simulink library "hose_pump_unit_v4"  (R2025b)
settings: Solver=VariableStepAuto  StartTime=0.0  StopTime=10.0  RelTol=1e-3
undefined symbols (not defined in the file): ACV_fit_coeffs, HP_bladder_elastic_modulus, HP_flowrate_damping_coefficient, HP_unstretched_fiber_angle, HP_unstretched_length, HP_unstretched_radius, HP_unstretched_wall_thickness, L_inlet, mu, power_avg_start_time, PTO_capacity_W, R_inlet, regulator_set_pressure_PSI, simu, SV_closing_threshold_Pa, SV_opening_threshold_Pa, turbine_gear_ratio
libraries: simulink x28, dspstat3 x4, turbine_generator_v0 x2, dsppolyfun x1, adjustable_check_valve_v0 x1
(part 1 of 2)
settings Model: Creator=Carson  LastModifiedBy=cmmcguir

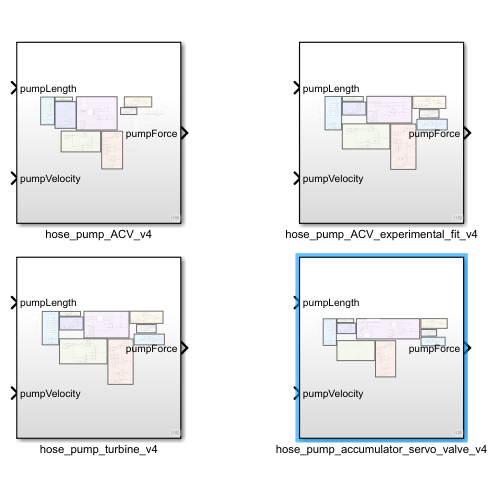
[thumbnail: Simulink's stored preview of the top-level diagram]
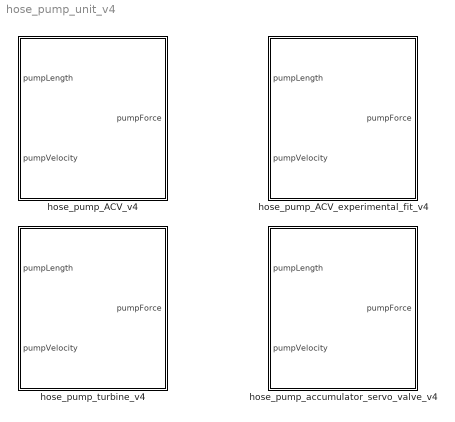
== system hose_pump_unit_v4 ==
  hose_pump_ACV_experimental_fit_v4 : Subsystem
  hose_pump_ACV_v4 : Subsystem
  hose_pump_accumulator_servo_valve_v4 : Subsystem
  hose_pump_turbine_v4 : Subsystem

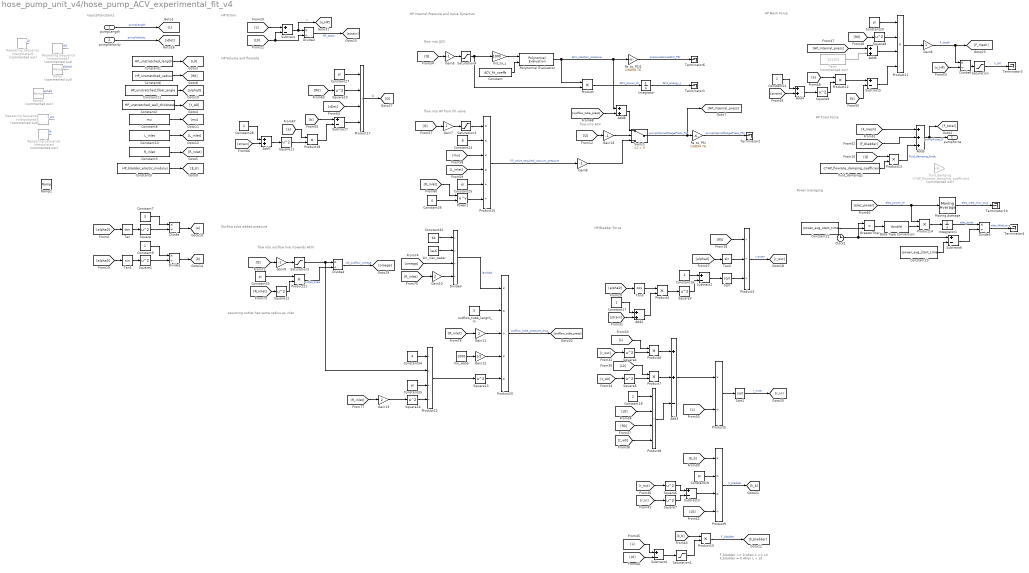
== system hose_pump_unit_v4/hose_pump_ACV_experimental_fit_v4 ==
  note: flow into ACV
  note: flow into ACV
  note: F_bladder >= 0 when L >= L0
      | F_bladder = 0 when L < L0
  note: HP Total Force
  note: HP Mesh Force
  note: HP Bladder Force
  note: HP Internal Pressure and Valve Dynamics
  note: HP Strain
  note: HP Volume and flowrate
  note: Inputs/Constants
  note: flow into HP from fill valve
  note: flow into outflow line (towards ACV)
  note: assuming outlet has same radius as inlet
  note: Outflow tube added pressure
  note: Power averaging
  pumpLength : Inport
  pumpVelocity : Inport  Port=2
  Add{2,4,6..8} (5 alike) : Sum
  Add3 : Sum  Inputs=++-
  Add5 : Sum  Inputs=+++
  Clock1 : Clock
  Constant : Constant  Value=ACV_fit_coeffs
  Constant1 : Constant  Value=HP_unstretched_length
  Constant10 : Constant  Value=L_inlet
  Constant11 : Constant  Value=HP_unstretched_fiber_angle
  Constant{9,16..17,21,28} (5 alike) : Constant
  Constant18 : Constant  Value=2
  Constant{19..20,25,27,33,35} (6 alike) : Constant  Value=pi
  Constant2 : Constant  Value=HP_unstretched_wall_thickness
  Constant22 : Constant  Value=power_avg_start_time
  Constant23 : Constant  Value=power_avg_start_time
  Constant24 : Constant  Value=8
  Constant26 : Constant  Value=4
  Constant3 : Constant  Value=R_inlet
  Constant32 : Constant  Value=64
  Constant34 : Constant  Value=4
  Constant5 : Constant  Value=HP_bladder_elastic_modulus
  Constant6 : Constant  Value=HP_unstretched_radius
  Constant7 : Constant  Value=3
  Constant8 : Constant  Value=mu
  Data Type Conversion : DataTypeConversion  OutDataTypeStr=double  SaturateOnIntegerOverflow=off  RndMeth=Floor
  Divide{,1..2,4..6} (6 alike) : Product  Inputs=*/
  Divide3 : Product  Inputs=**//
  Gain10 : Gain  Gain=2
  Gain11 : Gain  Gain=2
  Gain12 : Gain  Gain=1/2
  Gain13 : Gain  Gain=2
  Gain{5,8..9,14} (4 alike) : Gain  Gain=-1
  Gain6 : Gain
  Gain7 : Gain
  GreaterThan : RelationalOperator  Operator=>  OutDataTypeStr=boolean  RndMeth=Simplest  InputSameDT=off
  Integrator : Integrator
  Integrator1 : Integrator
  Moving Average : dspstat3/Moving Average  Method=Sliding window  ForgettingFactorPort=off  SpecifyWindowLength=on  WindowLength=30 / simu.dt  OverlapLength=30 / simu.dt - 1  AllowArbitraryInputLength=off  ForgettingFactor=0.9  SimulateUsing=Interpreted execution
  Pa_to_PSI : Gain  Gain=1/6894.76
  Pa_to_PSI1 : Gain  Gain=1/6894.76
  Patm : Constant  Commented=on  Value=101325
  Polynomial Evaluation : dsppolyfun/Polynomial Evaluation  useConstCoeffs=off  constCoeffs=[5 4 3 2 1]
  Power1 : Math  Operator=pow
  Product{,4,6..7,10,12..14,18,21} (10 alike) : Product
  Product11 : Product  Inputs=****
  Product15 : Product  Inputs=****//
  Product17 : Product  Inputs=****
  Product20 : Product  Inputs=**/**
  Product22 : Product  Inputs=**//
  Product3 : Product  Inputs=*/*
  Product5 : Product  Inputs=*/
  Product8 : Product  Inputs=****
  Product9 : Product  Inputs=***/
  Ramp : simulink/Sources/Ramp  Commented=on  slope=(1.25-1.12) / 2400  start=30  InitialOutput=1.12
  Ramp1 : simulink/Sources/Ramp  slope=5/1200  start=30  InitialOutput=1
  Ramp2 : simulink/Sources/Ramp  Commented=on  slope=(1.1 - 0.9) * HP_unstretched_fiber_angle / 2400  start=30  InitialOutput=0.9 * HP_unstretched_fiber_angle
  Repeating Sequence Interpolated : simulink/Sources/Repeating Sequence Interpolated  Commented=on  OutValues=HP_bladder_elastic_modulus * [0.75 2 0.75]  TimeValues=[0 60 120]*2  LookUpMeth=Interpolation-Use End Values  tsamp=simu.dt  OutMin=[]  OutMax=[]  OutDataTypeStr=double  OutputDataTypeScalingMode=double  OutDataType=fixdt(0,8)  OutScaling=2^-10
  Repeating Sequence Interpolated1 : simulink/Sources/Repeating Sequence Interpolated  Commented=on  OutValues=HP_unstretched_length * [0.8 1.2 0.8]  TimeValues=[0 60 120] * 4  LookUpMeth=Interpolation-Use End Values  tsamp=simu.dt  OutMin=[]  OutMax=[]  OutDataTypeStr=double  OutputDataTypeScalingMode=double  OutDataType=fixdt(0,8)  OutScaling=2^-10
  Repeating Sequence Interpolated2 : simulink/Sources/Repeating Sequence Interpolated  Commented=on  OutValues=HP_unstretched_radius * [0.8 1.2 0.8]  TimeValues=[0 60 120] * 4  LookUpMeth=Interpolation-Use End Values  tsamp=simu.dt  OutMin=[]  OutMax=[]  OutDataTypeStr=double  OutputDataTypeScalingMode=double  OutDataType=fixdt(0,8)  OutScaling=2^-10
  Repeating Sequence Interpolated3 : simulink/Sources/Repeating Sequence Interpolated  Commented=on  OutValues=HP_unstretched_wall_thickness * [0.75 1.25 0.75]  TimeValues=[0 60 120] * 4  LookUpMeth=Interpolation-Use End Values  tsamp=simu.dt  OutMin=[]  OutMax=[]  OutDataTypeStr=double  OutputDataTypeScalingMode=double  OutDataType=fixdt(0,8)  OutScaling=2^-10
  Saturation : Saturate  UpperLimit=10000  LowerLimit=-10000
  Saturation1 : Saturate  UpperLimit=inf  LowerLimit=0
  Saturation3 : Saturate  UpperLimit=inf  LowerLimit=0
  Saturation4 : Saturate  UpperLimit=inf  LowerLimit=0
  Saturation5 : Saturate  UpperLimit=inf  LowerLimit=1e-8
  Sqrt : Sqrt
  Sqrt1 : Sqrt
  Square{,1,3..14} (14 alike) : Math  Operator=square
  Subtract{,2..7} (7 alike) : Sum  Inputs=+-
  Switch : Switch  Criteria=u2 > Threshold  SaturateOnIntegerOverflow=off  InputSameDT=off
  Tan : Trigonometry  Operator=tan
  Tan1 : Trigonometry
  Tan2 : Trigonometry
  Tan3 : Trigonometry  Operator=cos
  Terminator{1..4,6,10} (6 alike) : Terminator
  fluid_damping : Gain  Commented=on  Gain=-1*HP_flowrate_damping_coefficient
  fluid_damping1 : Constant  Value=-1*HP_flowrate_damping_coefficient
  kin_visc_water : Constant  Value=1e-6
  m3_to_L : Gain  Gain=1000
  outflow_tube_length_m : Constant  Value=3
  rho_water : Constant  Value=1000
  pumpForce : Outport
  wires:
  [Q] -> Gain14/1
  [outflow_tube_press] -> Add8/2
  Constant2/1 -> [t_w0]
  Constant1/1 -> [L0]
  Constant5/1 -> [E_b]
  Constant11/1 -> [alpha0]
  pumpLength/1 -> [L]  "pumpLength"
  Constant6/1 -> [R0]
  Constant8/1 -> [mu]
  Constant10/1 -> [L_inlet]
  Switch/1 -> [HP_internal_press], Pa_to_PSI/1  "pumpInternalGuagePress_Pa"
  Pa_to_PSI/1 -> Terminator2/1  "pumpInternalGuagePress_PSI"
  Constant3/1 -> [R_inlet]
  Constant7/1 -> Divide/1
  [alpha0] -> Tan/1
  Tan/1 -> Square/1
  Square/1 -> Divide/2
  Divide/1 -> [a]
  Divide1/1 -> [b]
  Square1/1 -> Divide1/2
  Tan1/1 -> Square1/1
  [alpha0] -> Tan1/1
  Constant9/1 -> Divide1/1
  [L] -> Subtract/1
  [L0] -> Divide2/2, Subtract/2
  Subtract/1 -> [x_HP], Divide2/1  "x"
  Divide2/1 -> [strain]  "HP_strain"
  [R0] -> Product3/1
  [alpha0] -> Tan2/1
  Tan2/1 -> Product3/2
  Sqrt/1 -> Product3/3
  Subtract2/1 -> Sqrt/1
  Constant16/1 -> Subtract2/1
  [alpha0] -> Tan3/1
  Square3/1 -> Subtract2/2
  Product4/1 -> Square3/1
  Tan3/1 -> Product4/1
  Constant17/1 -> Add2/1
  [strain] -> Add2/2
  Add2/1 -> Product4/2
  Product3/1 -> [r_out]  "r_outer"
  Sqrt1/1 -> [r_in]  "r_inner"
  Product5/1 -> Sqrt1/1
  [L] -> Product5/2
  Add3/1 -> Product5/1
  Product6/1 -> Add3/1
  Square4/1 -> Product6/2
  [r_out] -> Square4/1
  [L] -> Product6/1
  [L0] -> Product7/1
  [t_w0] -> Square5/1
  Square5/1 -> Product7/2
  Product7/1 -> Add3/2
  Product8/1 -> Add3/3
  Constant18/1 -> Product8/1
  [L0] -> Product8/2
  [R0] -> Product8/3
  [t_w0] -> Product8/4
  [E_b] -> Product9/1
  Constant19/1 -> Product9/2
  Subtract3/1 -> Product9/3
  [r_out] -> Square6/1
  Square6/1 -> Subtract3/1
  [r_in] -> Square7/1
  Square7/1 -> Subtract3/2
  [L0] -> Product9/4
  Product9/1 -> [k_b]  "k_bladder"
  [k_b] -> Product10/1
  Subtract4/1 -> Saturation1/1
  [L0] -> Subtract4/2
  [L] -> Subtract4/1
  Product10/1 -> [F_bladder]  "F_bladder"
  [R0] -> Square8/1
  Constant20/1 -> Product11/1
  Square8/1 -> Product11/2
  [HP_internal_press] -> Add6/1
  [a] -> Product12/1
  Constant21/1 -> Add4/1
  Add4/1 -> Square9/1
  [strain] -> Add4/2
  Square9/1 -> Product12/2
  Product12/1 -> Subtract5/1
  [b] -> Subtract5/2
  Subtract5/1 -> Product11/4
  Gain6/1 -> Divide6/1, [F_mesh]  "F_mesh"
  Product13/1 -> Add5/3  "fluid_damping_force"
  Add5/1 -> [F_total], pumpForce/1  "pumpForce_N"
  Patm/1 -> Add6/2
  Add6/1 -> Product11/3
  [elec_power] -> Moving Average/1, Product14/1  "elec_power_W"
  Integrator1/1 -> Divide5/1  "elec_Joule"
  Divide5/1 -> Terminator4/1  "elec_Watt_avg"
  GreaterThan/1 -> Data Type Conversion/1
  Subtract6/1 -> Divide5/2
  Product14/1 -> Integrator1/1
  Constant23/1 -> Subtract6/2
  Constant22/1 -> GreaterThan/2
  Data Type Conversion/1 -> Product14/2
  Clock1/1 -> GreaterThan/1, Subtract6/1
  Saturation1/1 -> Product10/2
  [Q] -> Gain5/1
  Polynomial Evaluation/1 -> Product/1, Pa_to_PSI1/1, Add8/1  "ACV_reaction_pressure"
  [Q] -> Gain7/1
  Gain7/1 -> Saturation3/1
  Saturation3/1 -> Product15/1
  Constant24/1 -> Product15/2
  [mu] -> Product15/3
  [L_inlet] -> Product15/4
  Constant25/1 -> Product15/5
  Power1/1 -> Product15/6
  [R_inlet] -> Power1/1
  Constant26/1 -> Power1/2
  Product15/1 -> Gain8/1  "fill_valve_required_vacuum_pressure"
  Gain8/1 -> Switch/3
  Saturation4/1 -> Product/2, m3_to_L/1
  [F_mesh] -> Add5/1
  [F_bladder] -> Add5/2
  pumpVelocity/1 -> [xDot]  "pumpVelocity"
  Product17/1 -> [Q]  "Q"
  Square10/1 -> Product17/2
  Constant27/1 -> Product17/1
  [R0] -> Square10/1
  [xDot] -> Product17/3
  Subtract7/1 -> Product17/4
  [b] -> Subtract7/1
  Product18/1 -> Subtract7/2
  [strain] -> Add7/2
  Constant28/1 -> Add7/1
  Add7/1 -> Square11/1
  [a] -> Product18/1
  Square11/1 -> Product18/2
  Gain14/1 -> Switch/2
  Gain5/1 -> Saturation4/1
  Add8/1 -> Switch/1
  [R_inlet] -> Gain13/1
  Constant34/1 -> Product22/1
  Product20/1 -> [outflow_tube_press]  "outflow_tube_pressure_drop"
  Saturation5/1 -> Product22/2, Divide4/1
  Divide3/1 -> Product20/1  "lambda"
  rho_water/1 -> Gain12/1
  Constant35/1 -> Product22/3
  Square14/1 -> Product22/4
  [Q] -> Gain9/1
  kin_visc_water/1 -> Divide3/2
  Divide4/1 -> [omega]  "vel_outflow_omega"
  Gain10/1 -> Divide3/4
  Square13/1 -> Product20/5
  Product22/1 -> Square13/1
  [R_inlet] -> Gain11/1
  [R_inlet] -> Square12/1
  [R_inlet] -> Gain10/1
  Gain13/1 -> Square14/1
  Product21/1 -> Divide4/2  "outlet_area"
  Gain12/1 -> Product20/4
  [omega] -> Divide3/3
  Square12/1 -> Product21/2
  outflow_tube_length_m/1 -> Product20/2
  Gain11/1 -> Product20/3
  Gain9/1 -> Saturation5/1
  Constant33/1 -> Product21/1
  Constant32/1 -> Divide3/1
  [x_HP] -> Divide6/2
  Saturation/1 -> Terminator3/1  "k_HP"
  Divide6/1 -> Saturation/1
  Pa_to_PSI1/1 -> Terminator6/1  "pressureAcrossACV_PSI"
  Ramp/1 -> ?  "alpha0"
  Repeating Sequence Interpolated/1 -> ?  "Eb"
  Repeating Sequence Interpolated1/1 -> ?  "L0"
  Repeating Sequence Interpolated2/1 -> ?  "R0"
  Repeating Sequence Interpolated3/1 -> ?  "t_w0"
  [Q] -> Product13/1
  fluid_damping1/1 -> Product13/2
  Ramp2/1 -> ?  "alpha0"
  Product11/1 -> Gain6/1
  Moving Average/1 -> Terminator10/1  "elec_watt_mov_avg"
  Constant/1 -> Polynomial Evaluation/2
  m3_to_L/1 -> Polynomial Evaluation/1
  Product/1 -> Integrator/1  "ACV_power_W"
  Integrator/1 -> Terminator1/1  "ACV_energy_J"

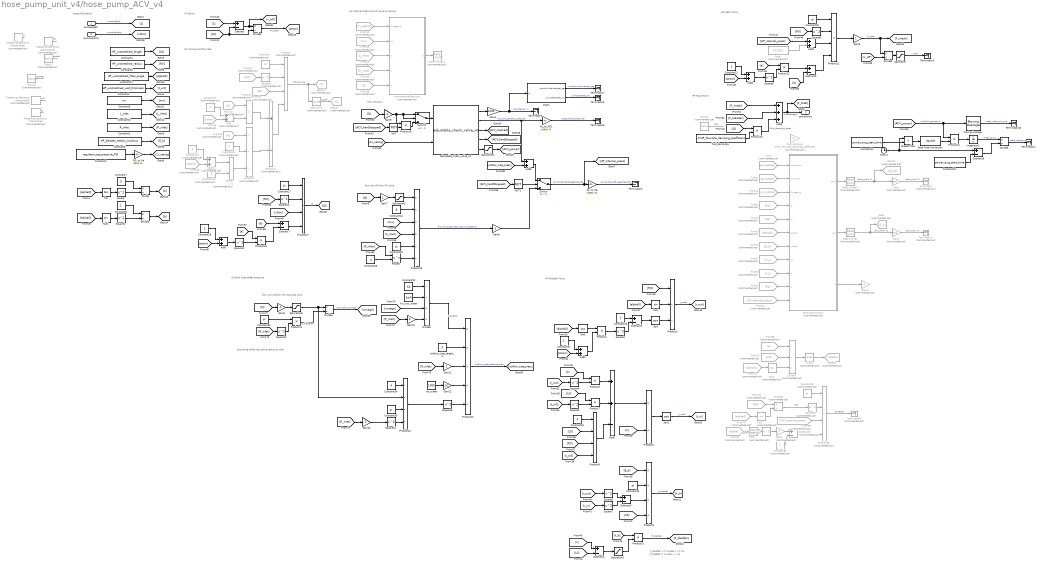
== system hose_pump_unit_v4/hose_pump_ACV_v4 ==
  note: flow into ACV
  note: F_bladder >= 0 when L >= L0
      | F_bladder = 0 when L < L0
  note: HP Total Force
  note: HP Mesh Force
  note: HP Bladder Force
  note: HP Internal Pressure and Valve Dynamics
  note: HP Strain
  note: HP Volume and flowrate
  note: Inputs/Constants
  note: flow into HP from fill valve
  note: flow into outflow line (towards ACV)
  note: assuming outlet has same radius as inlet
  note: Outflow tube added pressure
  pumpLength : Inport
  pumpVelocity : Inport  Port=2
  Acos : Trigonometry  Commented=on  Operator=acos
  Add : Sum  Commented=on
  Add1 : Sum  Commented=on
  Add{2,4,6..8} (5 alike) : Sum
  Add3 : Sum  Inputs=++-
  Add5 : Sum  Inputs=+++
  Chart : Stateflow chart  TreatAsAtomicUnit=on
  Clock1 : Clock
  Constant : Constant  Commented=on  Value=pi
  Constant1 : Constant  Value=HP_unstretched_length
  Constant10 : Constant  Value=L_inlet
  Constant11 : Constant  Value=HP_unstretched_fiber_angle
  Constant12 : Constant  Commented=on  Value=3
  Constant13 : Constant  Commented=on
  Constant14 : Constant  Commented=on
  Constant15 : Constant  Commented=on  Value=3
  Constant{9,16..17,21,28} (5 alike) : Constant
  Constant18 : Constant  Value=2
  Constant{19..20,25,27,33,35} (6 alike) : Constant  Value=pi
  Constant2 : Constant  Value=HP_unstretched_wall_thickness
  Constant22 : Constant  Value=power_avg_start_time
  Constant23 : Constant  Value=power_avg_start_time
  Constant24 : Constant  Value=8
  Constant26 : Constant  Value=4
  Constant29 : Constant  Commented=on  Value=pi
  Constant3 : Constant  Value=R_inlet
  Constant30 : Constant  Commented=on
  Constant32 : Constant  Value=64
  Constant34 : Constant  Value=4
  Constant4 : Constant  Value=regulator_set_pressure_PSI
  Constant5 : Constant  Value=HP_bladder_elastic_modulus
  Constant6 : Constant  Value=HP_unstretched_radius
  Constant7 : Constant  Value=3
  Constant8 : Constant  Value=mu
  Data Type Conversion : DataTypeConversion  OutDataTypeStr=double  SaturateOnIntegerOverflow=off  RndMeth=Floor
  Derivative : Derivative  Commented=on
  Divide{,1..2,4..6} (6 alike) : Product  Inputs=*/
  Divide3 : Product  Inputs=**//
  Divide7 : Product  Commented=on  Inputs=*/*
  Divide8 : Product  Commented=on  Inputs=*/
  From : From  Commented=on  GotoTag=pumpDisp
  From1 : From  Commented=on  GotoTag=pumpVel
  From11 : From  Commented=on  GotoTag=CV_setting
  From12 : From  Commented=on  GotoTag=CV_setting
  From13 : From  Commented=on  GotoTag=mu
  From14 : From  Commented=on  GotoTag=L_inlet
  From15 : From  Commented=on  GotoTag=R_inlet
  From16 : From  Commented=on  GotoTag=Q
  From17 : From  Commented=on  GotoTag=HP_internal_press
  From2 : From  Commented=on  GotoTag=R0
  From22 : From  Commented=on  GotoTag=R0
  From23 : From  Commented=on  GotoTag=L0
  From24 : From  Commented=on  GotoTag=b
  From25 : From  Commented=on  GotoTag=strain
  From26 : From  Commented=on  GotoTag=a
  From28 : From  Commented=on  GotoTag=strain
  From3 : From  Commented=on  GotoTag=L0
  From5 : From  Commented=on  GotoTag=alpha0
  From6 : From  Commented=on  GotoTag=E_b
  From69 : From  Commented=on  GotoTag=L
  From7 : From  Commented=on  GotoTag=mu
  From70 : From  Commented=on  GotoTag=L0
  From71 : From  Commented=on  GotoTag=alpha0
  From78 : From  Commented=on  GotoTag=R0
  From79 : From  Commented=on  GotoTag=alpha0
  From8 : From  Commented=on  GotoTag=Lt
  From80 : From  Commented=on  GotoTag=HP_internal_press
  From81 : From  Commented=on  GotoTag=alpha
  From9 : From  Commented=on  GotoTag=Rt
  Gain : Gain  Commented=on  Gain=1e6
  Gain1 : Gain  Commented=on  Gain=1e6
  Gain10 : Gain  Gain=2
  Gain11 : Gain  Gain=2
  Gain12 : Gain  Gain=1/2
  Gain13 : Gain  Gain=2
  Gain2 : Gain  Commented=on  Gain=-1
  Gain3 : Gain  Commented=on  Gain=3
  Gain4 : Gain  Gain=1000
  Gain5 : Gain  Gain=-1
  Gain6 : Gain
  Gain7 : Gain
  Gain8 : Gain  Gain=-1
  Gain9 : Gain  Gain=-1
  Goto : Goto  Commented=on  GotoTag=Q_in
  Goto13 : Goto  Commented=on  GotoTag=Q_out
  Goto16 : Goto  Commented=on  GotoTag=V
  Goto17 : Goto  Commented=on  GotoTag=Q
  Goto32 : Goto  Commented=on  GotoTag=alpha
  GreaterThan : RelationalOperator  Operator=>  OutDataTypeStr=boolean  RndMeth=Simplest  InputSameDT=off
  Integrator1 : Integrator
  MATLAB Function : MATLAB Function  Commented=on  TreatAsAtomicUnit=on
  Moving Average : dspstat3/Moving Average  Method=Sliding window  ForgettingFactorPort=off  SpecifyWindowLength=on  WindowLength=30 / simu.dt  OverlapLength=30 / simu.dt - 1  AllowArbitraryInputLength=off  ForgettingFactor=0.9  SimulateUsing=Interpreted execution
  NOT : Logic  Operator=NOT  IconShape=distinctive  AllPortsSameDT=off  OutDataTypeStr=boolean
  NOT1 : Logic  Operator=NOT  IconShape=distinctive  AllPortsSameDT=off  OutDataTypeStr=boolean
  PSI_to_Pa : Gain  Gain=6894.76
  Pa_to_PSI : Gain  Gain=1/6894.76
  Pa_to_PSI1 : Gain  Gain=1/6894.76
  Patm : Constant  Commented=on  Value=101325
  Power : Math  Commented=on  Operator=pow
  Power1 : Math  Operator=pow
  Product : Product  Commented=on  Inputs=****
  Product1 : Product  Commented=on  Inputs=**
  Product{4,6..7,10,12..14,16,18,21} (10 alike) : Product
  Product11 : Product  Inputs=****
  Product15 : Product  Inputs=****//
  Product17 : Product  Inputs=****
  Product19 : Product  Commented=on  Inputs=****
  Product2 : Product  Commented=on  Inputs=*/*
  Product20 : Product  Inputs=**/**
  Product22 : Product  Inputs=**//
  Product3 : Product  Inputs=*/*
  Product5 : Product  Inputs=*/
  Product8 : Product  Inputs=****
  Product9 : Product  Inputs=***/
  Ramp : simulink/Sources/Ramp  Commented=on  slope=(1.25-1.12) / 2400  start=30  InitialOutput=1.12
  Ramp1 : simulink/Sources/Ramp  Commented=on  slope=(1.2 - 0.8) * -1*HP_flowrate_damping_coefficient / 1200  start=30  InitialOutput=0.8 * -1*HP_flowrate_damping_coefficient
  Ramp2 : simulink/Sources/Ramp  Commented=on  slope=(1.1 - 0.9) * HP_unstretched_fiber_angle / 2400  start=30  InitialOutput=0.9 * HP_unstretched_fiber_angle
  Rate Limiter : RateLimiter  Commented=on  RisingSlewLimit=1e-3  FallingSlewLimit=-1e-3  SampleTimeMode=inherited
  Rate Limiter1 : RateLimiter  Commented=on  RisingSlewLimit=1e-3  FallingSlewLimit=-1e-3  SampleTimeMode=inherited
  Rate Limiter2 : RateLimiter  Commented=on  RisingSlewLimit=300*6894.76  FallingSlewLimit=-300*6894.76  SampleTimeMode=inherited
  Repeating Sequence Interpolated : simulink/Sources/Repeating Sequence Interpolated  Commented=on  OutValues=HP_bladder_elastic_modulus * [0.75 2 0.75]  TimeValues=[0 60 120]*2  LookUpMeth=Interpolation-Use End Values  tsamp=simu.dt  OutMin=[]  OutMax=[]  OutDataTypeStr=double  OutputDataTypeScalingMode=double  OutDataType=fixdt(0,8)  OutScaling=2^-10
  Repeating Sequence Interpolated1 : simulink/Sources/Repeating Sequence Interpolated  Commented=on  OutValues=HP_unstretched_length * [0.8 1.2 0.8]  TimeValues=[0 60 120] * 4  LookUpMeth=Interpolation-Use End Values  tsamp=simu.dt  OutMin=[]  OutMax=[]  OutDataTypeStr=double  OutputDataTypeScalingMode=double  OutDataType=fixdt(0,8)  OutScaling=2^-10
  Repeating Sequence Interpolated2 : simulink/Sources/Repeating Sequence Interpolated  Commented=on  OutValues=HP_unstretched_radius * [0.8 1.2 0.8]  TimeValues=[0 60 120] * 4  LookUpMeth=Interpolation-Use End Values  tsamp=simu.dt  OutMin=[]  OutMax=[]  OutDataTypeStr=double  OutputDataTypeScalingMode=double  OutDataType=fixdt(0,8)  OutScaling=2^-10
  Repeating Sequence Interpolated3 : simulink/Sources/Repeating Sequence Interpolated  Commented=on  OutValues=HP_unstretched_wall_thickness * [0.75 1.25 0.75]  TimeValues=[0 60 120] * 4  LookUpMeth=Interpolation-Use End Values  tsamp=simu.dt  OutMin=[]  OutMax=[]  OutDataTypeStr=double  OutputDataTypeScalingMode=double  OutDataType=fixdt(0,8)  OutScaling=2^-10
  Saturation : Saturate  UpperLimit=10000  LowerLimit=-10000
  Saturation1 : Saturate  UpperLimit=inf  LowerLimit=0
  Saturation2 : Saturate  UpperLimit=PTO_capacity_W  LowerLimit=0
  Saturation3 : Saturate  UpperLimit=inf  LowerLimit=0
  Saturation5 : Saturate  UpperLimit=inf  LowerLimit=1e-8
  Sqrt : Sqrt
  Sqrt1 : Sqrt
  Square{,1,3..14} (14 alike) : Math  Operator=square
  Square15 : Math  Commented=on  Operator=square
  Square16 : Math  Commented=on  Operator=square
  Square2 : Math  Commented=on  Operator=square
  Subtract{,2..7} (7 alike) : Sum  Inputs=+-
  Subtract1 : Sum  Commented=on  Inputs=+-
  Subtract8 : Sum  Commented=on  Inputs=+-
  Switch : Switch  Criteria=u2 > Threshold  SaturateOnIntegerOverflow=off  InputSameDT=off
  Switch1 : Switch  Criteria=u2 > Threshold  SaturateOnIntegerOverflow=off  InputSameDT=off
  Tan : Trigonometry  Operator=tan
  Tan1 : Trigonometry
  Tan2 : Trigonometry
  Tan3 : Trigonometry  Operator=cos
  Tan4 : Trigonometry  Commented=on  Operator=cos
  Tan5 : Trigonometry  Commented=on
  Tan6 : Trigonometry  Commented=on  Operator=cos
  Terminator : Terminator  Commented=on
  Terminator1 : Terminator  Commented=on
  Terminator{2..8,10} (8 alike) : Terminator
  Terminator9 : Terminator  Commented=on
  adjustable_check_valve_v0 : adjustable_check_valve_v0/adjustable_check_valve_v0  SystemSampleTime=-1  VariantActivationTime=update diagram  EmptyChoice=off  PassThrough=off  PassThroughVariantControl=(default)  EmptyChoiceVariantControl=(default)  AllowFlexibleInterface=on  Latency=0  AutoFrameSizeCalculation=off
  fluid_damping : Gain  Commented=on  Gain=-1*HP_flowrate_damping_coefficient
  fluid_damping1 : Constant  Value=-1*HP_flowrate_damping_coefficient
  kin_visc_water : Constant  Value=1e-6
  outflow_tube_length_m : Constant  Value=3
  pumpInternalPressure : MATLAB Function  Commented=on  TreatAsAtomicUnit=on
  rho_water : Constant  Value=1000
  pumpForce : Outport
  wires:
  [outflow_tube_press] -> Add8/2
  Constant2/1 -> [t_w0]
  Constant1/1 -> [L0]
  Constant5/1 -> [E_b]
  Constant11/1 -> [alpha0]
  pumpLength/1 -> [L]  "pumpLength"
  Constant6/1 -> [R0]
  Constant8/1 -> [mu]
  Constant10/1 -> [L_inlet]
  From/1 -> MATLAB Function/1(pumpDisp)
  From1/1 -> MATLAB Function/2(pumpVel)
  From2/1 -> MATLAB Function/4(r0)
  From3/1 -> MATLAB Function/5(L0)
  From5/1 -> MATLAB Function/6(alpha0)
  From6/1 -> MATLAB Function/7(k_tube)
  From7/1 -> MATLAB Function/8(mu)
  From8/1 -> MATLAB Function/9(lt)
  From9/1 -> MATLAB Function/10(rt)
  Rate Limiter1/1 -> Goto13/1, Gain/1  "Qout_m3-s^-1"
  Rate Limiter/1 -> Goto/1, Gain1/1  "Qin_m3-s^-1"
  Switch/1 -> [HP_internal_press], Pa_to_PSI/1  "pumpInternalGuagePress_Pa"
  From11/1 -> MATLAB Function/3(CV_setting)
  Gain/1 -> Terminator/1  "Qout_mL-s^-1"
  Gain1/1 -> Terminator1/1  "Qin_mL-s^-1"
  Pa_to_PSI/1 -> Terminator2/1  "pumpInternalGuagePress_PSI"
  MATLAB Function/3(F) -> Gain2/1
  Constant4/1 -> PSI_to_Pa/1
  PSI_to_Pa/1 -> [CV_setting]
  From12/1 -> pumpInternalPressure/1(CV_setting)
  From13/1 -> pumpInternalPressure/2(mu)
  From14/1 -> pumpInternalPressure/3(lt)
  From15/1 -> pumpInternalPressure/4(rt)
  From16/1 -> pumpInternalPressure/5(Q)
  From17/1 -> MATLAB Function/11(P)
  pumpInternalPressure/1(P) -> Rate Limiter2/1
  MATLAB Function/2(Qin) -> Rate Limiter/1
  MATLAB Function/1(Qout) -> Rate Limiter1/1
  Constant3/1 -> [R_inlet]
  Constant7/1 -> Divide/1
  [alpha0] -> Tan/1
  Tan/1 -> Square/1
  Square/1 -> Divide/2
  Divide/1 -> [a]
  Divide1/1 -> [b]
  Square1/1 -> Divide1/2
  Tan1/1 -> Square1/1
  [alpha0] -> Tan1/1
  Constant9/1 -> Divide1/1
  [L] -> Subtract/1
  [L0] -> Divide2/2, Subtract/2
  Subtract/1 -> [x_HP], Divide2/1  "x"
  Divide2/1 -> [strain]  "HP_strain"
  From22/1 -> Square2/1
  Constant/1 -> Product/1
  Square2/1 -> Product/2
  From23/1 -> Product/3
  Constant12/1 -> Product2/2
  From24/1 -> Product1/1
  From25/1 -> Add/2
  Constant13/1 -> Add/1
  Add/1 -> Product1/2
  Product1/1 -> Subtract1/1
  Subtract1/1 -> Product/4
  Product2/1 -> Subtract1/2
  From26/1 -> Product2/1
  Constant14/1 -> Add1/1
  From28/1 -> Add1/2
  Power/1 -> Product2/3
  Add1/1 -> Power/1
  Constant15/1 -> Power/2
  Product/1 -> Derivative/1, Goto16/1  "HP_volume"
  Derivative/1 -> Goto17/1  "Q_old"
  [R0] -> Product3/1
  [alpha0] -> Tan2/1
  Tan2/1 -> Product3/2
  Sqrt/1 -> Product3/3
  Subtract2/1 -> Sqrt/1
  Constant16/1 -> Subtract2/1
  [alpha0] -> Tan3/1
  Square3/1 -> Subtract2/2
  Product4/1 -> Square3/1
  Tan3/1 -> Product4/1
  Constant17/1 -> Add2/1
  [strain] -> Add2/2
  Add2/1 -> Product4/2
  Product3/1 -> [r_out]  "r_outer"
  Sqrt1/1 -> [r_in]  "r_inner"
  Product5/1 -> Sqrt1/1
  [L] -> Product5/2
  Add3/1 -> Product5/1
  Product6/1 -> Add3/1
  Square4/1 -> Product6/2
  [r_out] -> Square4/1
  [L] -> Product6/1
  [L0] -> Product7/1
  [t_w0] -> Square5/1
  Square5/1 -> Product7/2
  Product7/1 -> Add3/2
  Product8/1 -> Add3/3
  Constant18/1 -> Product8/1
  [L0] -> Product8/2
  [R0] -> Product8/3
  [t_w0] -> Product8/4
  [E_b] -> Product9/1
  Constant19/1 -> Product9/2
  Subtract3/1 -> Product9/3
  [r_out] -> Square6/1
  Square6/1 -> Subtract3/1
  [r_in] -> Square7/1
  Square7/1 -> Subtract3/2
  [L0] -> Product9/4
  Product9/1 -> [k_b]  "k_bladder"
  [k_b] -> Product10/1
  Subtract4/1 -> Saturation1/1
  [L0] -> Subtract4/2
  [L] -> Subtract4/1
  Product10/1 -> [F_bladder]  "F_bladder"
  [R0] -> Square8/1
  Constant20/1 -> Product11/1
  Square8/1 -> Product11/2
  [HP_internal_press] -> Add6/1
  [a] -> Product12/1
  Constant21/1 -> Add4/1
  Add4/1 -> Square9/1
  [strain] -> Add4/2
  Square9/1 -> Product12/2
  Product12/1 -> Subtract5/1
  [b] -> Subtract5/2
  Subtract5/1 -> Product11/4
  Gain6/1 -> Divide6/1, [F_mesh]  "F_mesh"
  Product13/1 -> Add5/3  "fluid_damping_force"
  Add5/1 -> [F_total], pumpForce/1  "pumpForce_N"
  Patm/1 -> Add6/2
  Add6/1 -> Product11/3
  [ACV_power] -> Moving Average/1, Product14/1  "hydraulic_power_W"
  Integrator1/1 -> Divide5/1  "mech_Joule"
  Divide5/1 -> Terminator4/1  "mech_Watt_avg"
  GreaterThan/1 -> Data Type Conversion/1
  Subtract6/1 -> Divide5/2
  Product14/1 -> Integrator1/1
  Constant23/1 -> Subtract6/2
  Constant22/1 -> GreaterThan/2
  Data Type Conversion/1 -> Product14/2
  Clock1/1 -> GreaterThan/1, Subtract6/1
  Saturation1/1 -> Product10/2
  [Q] -> Gain5/1
  [CV_setting] -> adjustable_check_valve_v0/2
  adjustable_check_valve_v0/1 -> Gain4/1
  adjustable_check_valve_v0/2 -> Pa_to_PSI1/1, Add8/1  "ACV_disk_reaction_pressure"
  [Q] -> Gain7/1
  Gain7/1 -> Saturation3/1
  Saturation3/1 -> Product15/1
  Constant24/1 -> Product15/2
  [mu] -> Product15/3
  [L_inlet] -> Product15/4
  Constant25/1 -> Product15/5
  Power1/1 -> Product15/6
  [R_inlet] -> Power1/1
  Constant26/1 -> Power1/2
  Product15/1 -> Gain8/1  "fill_valve_required_vacuum_pressure"
  Gain8/1 -> Switch/3
  adjustable_check_valve_v0/3 -> [ACV_cracked]
  Switch1/1 -> adjustable_check_valve_v0/1
  adjustable_check_valve_v0/5 -> Saturation2/1
  [F_mesh] -> Add5/1
  [F_bladder] -> Add5/2
  pumpVelocity/1 -> [xDot]  "pumpVelocity"
  Product17/1 -> [Q]  "Q"
  Square10/1 -> Product17/2
  Constant27/1 -> Product17/1
  [R0] -> Square10/1
  [xDot] -> Product17/3
  Subtract7/1 -> Product17/4
  [b] -> Subtract7/1
  Product18/1 -> Subtract7/2
  [strain] -> Add7/2
  Constant28/1 -> Add7/1
  Add7/1 -> Square11/1
  [a] -> Product18/1
  Square11/1 -> Product18/2
  NOT1/1 -> Switch/2
  adjustable_check_valve_v0/4 -> [ACV_hardStopped]
  [ACV_hardStopped] -> NOT/1
  NOT/1 -> Product16/2
  Gain5/1 -> Product16/1, Switch1/2, Switch1/1
  Product16/1 -> Switch1/3
  [ACV_hardStopped] -> NOT1/1
  Add8/1 -> Switch/1
  [R_inlet] -> Gain13/1
  Constant34/1 -> Product22/1
  Product20/1 -> [outflow_tube_press]  "outflow_tube_pressure_drop"
  Saturation5/1 -> Product22/2, Divide4/1
  Divide3/1 -> Product20/1  "lambda"
  rho_water/1 -> Gain12/1
  Constant35/1 -> Product22/3
  Square14/1 -> Product22/4
  [Q] -> Gain9/1
  kin_visc_water/1 -> Divide3/2
  Divide4/1 -> [omega]  "vel_outflow_omega"
  Gain10/1 -> Divide3/4
  Square13/1 -> Product20/5
  Product22/1 -> Square13/1
  [R_inlet] -> Gain11/1
  [R_inlet] -> Square12/1
  [R_inlet] -> Gain10/1
  Gain13/1 -> Square14/1
  Product21/1 -> Divide4/2  "outlet_area"
  Gain12/1 -> Product20/4
  [omega] -> Divide3/3
  Square12/1 -> Product21/2
  outflow_tube_length_m/1 -> Product20/2
  Gain11/1 -> Product20/3
  Gain9/1 -> Saturation5/1
  Constant33/1 -> Product21/1
  Constant32/1 -> Divide3/1
  [x_HP] -> Divide6/2
  Saturation/1 -> Terminator3/1  "k_HP"
  Divide6/1 -> Saturation/1
  Gain4/1 -> Chart/1(Q), Terminator5/1  "Q_outlet_Ls^-1"
  Pa_to_PSI1/1 -> Terminator6/1  "pressureAcrossACV_PSI"
  Ramp/1 -> ?  "alpha0"
  Repeating Sequence Interpolated/1 -> ?  "Eb"
  Chart/1(pumpWindowLength_sec) -> Terminator7/1  "pumpWindowLength_sec"
  Repeating Sequence Interpolated1/1 -> ?  "L0"
  Repeating Sequence Interpolated2/1 -> ?  "R0"
  Repeating Sequence Interpolated3/1 -> ?  "t_w0"
  Chart/2(pumpedWater_mL) -> Terminator8/1  "pumpedWater_mL"
  [Q] -> Product13/1
  Ramp1/1 -> ?  "C_Q"
  fluid_damping1/1 -> Product13/2
  Ramp2/1 -> ?  "alpha0"
  From71/1 -> Tan4/1
  From69/1 -> Divide7/1
  From70/1 -> Divide7/2
  Tan4/1 -> Divide7/3
  Divide7/1 -> Acos/1
  Acos/1 -> Goto32/1
  Tan5/1 -> Divide8/2
  From79/1 -> Tan5/1
  From78/1 -> Divide8/1
  Divide8/1 -> Square15/1  "r90"
  Constant29/1 -> Product19/1
  Square15/1 -> Product19/2
  From80/1 -> Product19/3
  From81/1 -> Tan6/1
  Tan6/1 -> Square16/1
  Square16/1 -> Gain3/1
  Gain3/1 -> Subtract8/1
  Constant30/1 -> Subtract8/2
  Subtract8/1 -> Product19/4
  Product19/1 -> Terminator9/1  "F_mesh2"
  Product11/1 -> Gain6/1
  Moving Average/1 -> Terminator10/1  "mech_watt_mov_avg"
  Saturation2/1 -> [ACV_power]

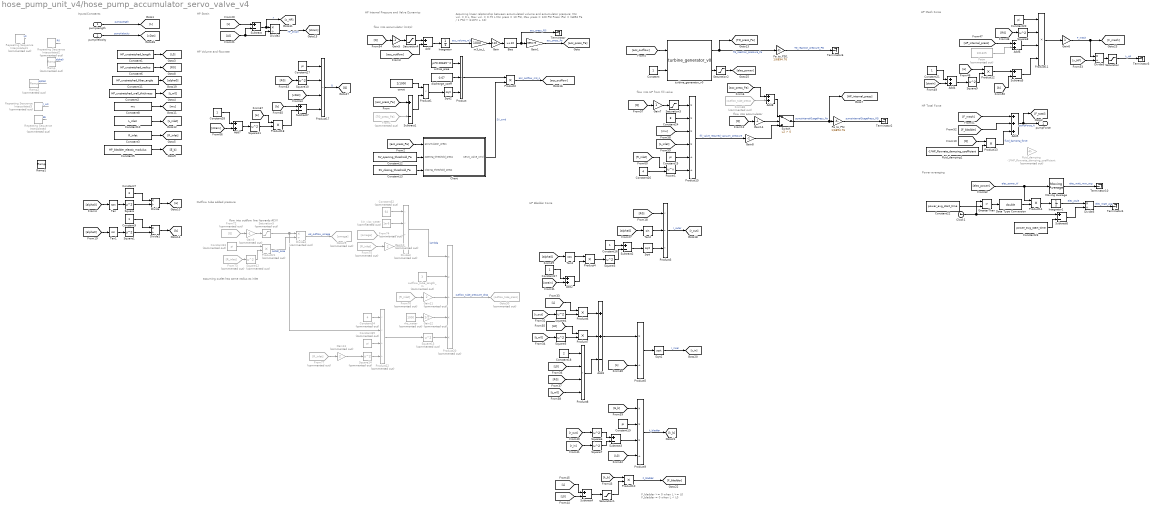
== system hose_pump_unit_v4/hose_pump_accumulator_servo_valve_v4 ==
  note: Assuming linear relationship between accumulated volume and accumulator pressure:
      |  Min vol. = 0 L,   Max vol. = 0.75 L
      |  Min press = 10 PSI,   Max press = 120 PSI
      |  Press (Pa) = (6894 Pa / 1 PSI) * (110*V + 10)
  note: flow into accumulator
  note: flow into accumulator (m3/s)
  note: F_bladder >= 0 when L >= L0
      | F_bladder = 0 when L < L0
  note: HP Total Force
  note: HP Mesh Force
  note: HP Bladder Force
  note: HP Internal Pressure and Valve Dynamics
  note: HP Strain
  note: HP Volume and flowrate
  note: Inputs/Constants
  note: flow into HP from fill valve
  note: flow into outflow line (towards ACV)
  note: assuming outlet has same radius as inlet
  note: Outflow tube added pressure
  note: Power averaging
  pumpLength : Inport
  pumpVelocity : Inport  Port=2
  Add : Sum  Inputs=+-
  Add{2,4,6..8} (5 alike) : Sum
  Add3 : Sum  Inputs=++-
  Add5 : Sum  Inputs=+++
  Bias : Bias  Bias=10  SaturateOnIntegerOverflow=off
  Chart : Stateflow chart  TreatAsAtomicUnit=on
  Clock1 : Clock
  Constant{,9,16..17,21,28} (6 alike) : Constant
  Constant1 : Constant  Value=HP_unstretched_length
  Constant10 : Constant  Value=L_inlet
  Constant11 : Constant  Value=HP_unstretched_fiber_angle
  Constant12 : Constant  Value=SV_opening_threshold_Pa
  Constant13 : Constant  Value=SV_closing_threshold_Pa
  Constant18 : Constant  Value=2
  Constant{19..20,25,27} (4 alike) : Constant  Value=pi
  Constant2 : Constant  Value=HP_unstretched_wall_thickness
  Constant22 : Constant  Value=power_avg_start_time
  Constant23 : Constant  Value=power_avg_start_time
  Constant24 : Constant  Value=8
  Constant26 : Constant  Value=4
  Constant3 : Constant  Value=R_inlet
  Constant32 : Constant  Commented=on  Value=64
  Constant33 : Constant  Commented=on  Value=pi
  Constant34 : Constant  Commented=on  Value=4
  Constant35 : Constant  Commented=on  Value=pi
  Constant5 : Constant  Value=HP_bladder_elastic_modulus
  Constant6 : Constant  Value=HP_unstretched_radius
  Constant7 : Constant  Value=3
  Constant8 : Constant  Value=mu
  Data Type Conversion : DataTypeConversion  OutDataTypeStr=double  SaturateOnIntegerOverflow=off  RndMeth=Floor
  Divide{,1..2,5..6} (5 alike) : Product  Inputs=*/
  Divide3 : Product  Commented=on  Inputs=**//
  Divide4 : Product  Commented=on  Inputs=*/
  From1 : From  Commented=on  GotoTag=TG_press_Pa
  From68 : From  Commented=on  GotoTag=outflow_tube_press
  From72 : From  Commented=on  GotoTag=Q
  From{73,75..77} (4 alike) : From  Commented=on  GotoTag=R_inlet
  From74 : From  Commented=on  GotoTag=omega
  Gain : Gain  Gain=110
  Gain1 : Gain  Gain=6894.76
  Gain10 : Gain  Commented=on  Gain=2
  Gain11 : Gain  Commented=on  Gain=2
  Gain12 : Gain  Commented=on  Gain=1/2
  Gain13 : Gain  Commented=on  Gain=2
  Gain14 : Gain  Gain=-1
  Gain5 : Gain  Gain=-1
  Gain6 : Gain
  Gain7 : Gain
  Gain8 : Gain  Gain=-1
  Gain9 : Gain  Commented=on  Gain=-1
  Goto29 : Goto  Commented=on  GotoTag=omega
  Goto30 : Goto  Commented=on  GotoTag=outflow_tube_press
  GreaterThan : RelationalOperator  Operator=>  OutDataTypeStr=boolean  RndMeth=Simplest  InputSameDT=off
  Integrator : Integrator
  Integrator1 : Integrator
  Moving Average : dspstat3/Moving Average  Method=Sliding window  ForgettingFactorPort=off  SpecifyWindowLength=on  WindowLength=30 / simu.dt  OverlapLength=30 / simu.dt - 1  AllowArbitraryInputLength=off  ForgettingFactor=0.9  SimulateUsing=Interpreted execution
  Pa_to_PSI : Gain  Gain=1/6894.76
  Pa_to_PSI1 : Gain  Gain=1/6894.76
  Patm : Constant  Commented=on  Value=101325
  Power1 : Math  Operator=pow
  Product : Product  Inputs=***
  Product{1..2,4,6..7,10,12..14,18} (10 alike) : Product
  Product11 : Product  Inputs=****
  Product15 : Product  Inputs=****//
  Product17 : Product  Inputs=****
  Product20 : Product  Commented=on  Inputs=**/**
  Product21 : Product  Commented=on
  Product22 : Product  Commented=on  Inputs=**//
  Product3 : Product  Inputs=*/*
  Product5 : Product  Inputs=*/
  Product8 : Product  Inputs=****
  Product9 : Product  Inputs=***/
  Ramp : simulink/Sources/Ramp  Commented=on  slope=(1.25-1.12) / 2400  start=30  InitialOutput=1.12
  Ramp1 : simulink/Sources/Ramp  slope=5/1200  start=30  InitialOutput=1
  Ramp2 : simulink/Sources/Ramp  Commented=on  slope=(1.1 - 0.9) * HP_unstretched_fiber_angle / 2400  start=30  InitialOutput=0.9 * HP_unstretched_fiber_angle
  Repeating Sequence Interpolated : simulink/Sources/Repeating Sequence Interpolated  Commented=on  OutValues=HP_bladder_elastic_modulus * [0.75 2 0.75]  TimeValues=[0 60 120]*2  LookUpMeth=Interpolation-Use End Values  tsamp=simu.dt  OutMin=[]  OutMax=[]  OutDataTypeStr=double  OutputDataTypeScalingMode=double  OutDataType=fixdt(0,8)  OutScaling=2^-10
  Repeating Sequence Interpolated1 : simulink/Sources/Repeating Sequence Interpolated  Commented=on  OutValues=HP_unstretched_length * [0.8 1.2 0.8]  TimeValues=[0 60 120] * 4  LookUpMeth=Interpolation-Use End Values  tsamp=simu.dt  OutMin=[]  OutMax=[]  OutDataTypeStr=double  OutputDataTypeScalingMode=double  OutDataType=fixdt(0,8)  OutScaling=2^-10
  Repeating Sequence Interpolated2 : simulink/Sources/Repeating Sequence Interpolated  Commented=on  OutValues=HP_unstretched_radius * [0.8 1.2 0.8]  TimeValues=[0 60 120] * 4  LookUpMeth=Interpolation-Use End Values  tsamp=simu.dt  OutMin=[]  OutMax=[]  OutDataTypeStr=double  OutputDataTypeScalingMode=double  OutDataType=fixdt(0,8)  OutScaling=2^-10
  Repeating Sequence Interpolated3 : simulink/Sources/Repeating Sequence Interpolated  Commented=on  OutValues=HP_unstretched_wall_thickness * [0.75 1.25 0.75]  TimeValues=[0 60 120] * 4  LookUpMeth=Interpolation-Use End Values  tsamp=simu.dt  OutMin=[]  OutMax=[]  OutDataTypeStr=double  OutputDataTypeScalingMode=double  OutDataType=fixdt(0,8)  OutScaling=2^-10
  Saturation : Saturate  UpperLimit=10000  LowerLimit=-10000
  Saturation1 : Saturate  UpperLimit=inf  LowerLimit=0
  Saturation2 : Saturate  UpperLimit=PTO_capacity_W  LowerLimit=-inf
  Saturation3 : Saturate  UpperLimit=inf  LowerLimit=0
  Saturation4 : Saturate  UpperLimit=inf  LowerLimit=0
  Saturation5 : Saturate  Commented=on  UpperLimit=inf  LowerLimit=1e-8
  Sqrt : Sqrt
  Sqrt1 : Sqrt
  Sqrt2 : Sqrt
  Square{,1,3..11} (11 alike) : Math  Operator=square
  Square12 : Math  Commented=on  Operator=square
  Square13 : Math  Commented=on  Operator=square
  Square14 : Math  Commented=on  Operator=square
  Subtract{,1..7} (8 alike) : Sum  Inputs=+-
  Switch : Switch  Criteria=u2 > Threshold  SaturateOnIntegerOverflow=off  InputSameDT=off
  Tan : Trigonometry  Operator=tan
  Tan1 : Trigonometry
  Tan2 : Trigonometry
  Tan3 : Trigonometry  Operator=cos
  Terminator{,2..4,6,10} (6 alike) : Terminator
  const : Constant  Value=2/1000
  discharge_coeff : Constant  Value=0.67
  fluid_damping : Gain  Commented=on  Gain=-1*HP_flowrate_damping_coefficient
  fluid_damping1 : Constant  Value=-1*HP_flowrate_damping_coefficient
  kin_visc_water : Constant  Commented=on  Value=1e-6
  m3_to_L : Gain  Gain=1000
  orifice_area : Constant  Value=pi*0.00635^2
  outflow_tube_length_m : Constant  Commented=on  Value=3
  rho_water : Constant  Commented=on  Value=1000
  turbine_generator_v0 : turbine_generator_v0/turbine_generator_v0  SystemSampleTime=-1  VariantActivationTime=update diagram  EmptyChoice=off  PassThrough=off  PassThroughVariantControl=(default)  EmptyChoiceVariantControl=(default)  AllowFlexibleInterface=on  Latency=0  AutoFrameSizeCalculation=off
  pumpForce : Outport
  wires:
  [Q] -> Gain14/1
  From68/1 -> Add8/2
  Constant2/1 -> [t_w0]
  Constant1/1 -> [L0]
  Constant5/1 -> [E_b]
  Constant11/1 -> [alpha0]
  pumpLength/1 -> [L]  "pumpLength"
  Constant6/1 -> [R0]
  Constant8/1 -> [mu]
  Constant10/1 -> [L_inlet]
  Switch/1 -> [HP_internal_press], Pa_to_PSI/1  "pumpInternalGuagePress_Pa"
  Pa_to_PSI/1 -> Terminator2/1  "pumpInternalGuagePress_PSI"
  Constant3/1 -> [R_inlet]
  Constant7/1 -> Divide/1
  [alpha0] -> Tan/1
  Tan/1 -> Square/1
  Square/1 -> Divide/2
  Divide/1 -> [a]
  Divide1/1 -> [b]
  Square1/1 -> Divide1/2
  Tan1/1 -> Square1/1
  [alpha0] -> Tan1/1
  Constant9/1 -> Divide1/1
  [L] -> Subtract/1
  [L0] -> Divide2/2, Subtract/2
  Subtract/1 -> [x_HP], Divide2/1  "x"
  Divide2/1 -> [strain]  "HP_strain"
  [R0] -> Product3/1
  [alpha0] -> Tan2/1
  Tan2/1 -> Product3/2
  Sqrt/1 -> Product3/3
  Subtract2/1 -> Sqrt/1
  Constant16/1 -> Subtract2/1
  [alpha0] -> Tan3/1
  Square3/1 -> Subtract2/2
  Product4/1 -> Square3/1
  Tan3/1 -> Product4/1
  Constant17/1 -> Add2/1
  [strain] -> Add2/2
  Add2/1 -> Product4/2
  Product3/1 -> [r_out]  "r_outer"
  Sqrt1/1 -> [r_in]  "r_inner"
  Product5/1 -> Sqrt1/1
  [L] -> Product5/2
  Add3/1 -> Product5/1
  Product6/1 -> Add3/1
  Square4/1 -> Product6/2
  [r_out] -> Square4/1
  [L] -> Product6/1
  [L0] -> Product7/1
  [t_w0] -> Square5/1
  Square5/1 -> Product7/2
  Product7/1 -> Add3/2
  Product8/1 -> Add3/3
  Constant18/1 -> Product8/1
  [L0] -> Product8/2
  [R0] -> Product8/3
  [t_w0] -> Product8/4
  [E_b] -> Product9/1
  Constant19/1 -> Product9/2
  Subtract3/1 -> Product9/3
  [r_out] -> Square6/1
  Square6/1 -> Subtract3/1
  [r_in] -> Square7/1
  Square7/1 -> Subtract3/2
  [L0] -> Product9/4
  Product9/1 -> [k_b]  "k_bladder"
  [k_b] -> Product10/1
  Subtract4/1 -> Saturation1/1
  [L0] -> Subtract4/2
  [L] -> Subtract4/1
  Product10/1 -> [F_bladder]  "F_bladder"
  [R0] -> Square8/1
  Constant20/1 -> Product11/1
  Square8/1 -> Product11/2
  [HP_internal_press] -> Add6/1
  [a] -> Product12/1
  Constant21/1 -> Add4/1
  Add4/1 -> Square9/1
  [strain] -> Add4/2
  Square9/1 -> Product12/2
  Product12/1 -> Subtract5/1
  [b] -> Subtract5/2
  Subtract5/1 -> Product11/4
  Gain6/1 -> Divide6/1, [F_mesh]  "F_mesh"
  Product13/1 -> Add5/3  "fluid_damping_force"
  Add5/1 -> [F_total], pumpForce/1  "pumpForce_N"
  Patm/1 -> Add6/2
  Add6/1 -> Product11/3
  [elec_power] -> Moving Average/1, Product14/1  "elec_power_W"
  Integrator1/1 -> Divide5/1  "elec_Joule"
  Divide5/1 -> Terminator4/1  "elec_Watt_avg"
  GreaterThan/1 -> Data Type Conversion/1
  Subtract6/1 -> Divide5/2
  Product14/1 -> Integrator1/1
  Constant23/1 -> Subtract6/2
  Constant22/1 -> GreaterThan/2
  Data Type Conversion/1 -> Product14/2
  Clock1/1 -> GreaterThan/1, Subtract6/1
  Saturation1/1 -> Product10/2
  [Q] -> Gain5/1
  Constant/1 -> turbine_generator_v0/2
  turbine_generator_v0/1 -> [TG_press_Pa], Pa_to_PSI1/1  "TG_reaction_pressure_Pa"
  [Q] -> Gain7/1
  Gain7/1 -> Saturation3/1
  Saturation3/1 -> Product15/1
  Constant24/1 -> Product15/2
  [mu] -> Product15/3
  [L_inlet] -> Product15/4
  Constant25/1 -> Product15/5
  Power1/1 -> Product15/6
  [R_inlet] -> Power1/1
  Constant26/1 -> Power1/2
  Product15/1 -> Gain8/1  "fill_valve_required_vacuum_pressure"
  Gain8/1 -> Switch/3
  Saturation4/1 -> Add/1
  turbine_generator_v0/2 -> Saturation2/1
  [F_mesh] -> Add5/1
  [F_bladder] -> Add5/2
  pumpVelocity/1 -> [xDot]  "pumpVelocity"
  Product17/1 -> [Q]  "Q"
  Square10/1 -> Product17/2
  Constant27/1 -> Product17/1
  [R0] -> Square10/1
  [xDot] -> Product17/3
  Subtract7/1 -> Product17/4
  [b] -> Subtract7/1
  Product18/1 -> Subtract7/2
  [strain] -> Add7/2
  Constant28/1 -> Add7/1
  Add7/1 -> Square11/1
  [a] -> Product18/1
  Square11/1 -> Product18/2
  Gain14/1 -> Switch/2
  Gain5/1 -> Saturation4/1
  Add8/1 -> Switch/1
  From77/1 -> Gain13/1
  Constant34/1 -> Product22/1
  Product20/1 -> Goto30/1  "outflow_tube_pressure_drop"
  Saturation5/1 -> Product22/2, Divide4/1
  Divide3/1 -> Product20/1  "lambda"
  rho_water/1 -> Gain12/1
  Constant35/1 -> Product22/3
  Square14/1 -> Product22/4
  From72/1 -> Gain9/1
  kin_visc_water/1 -> Divide3/2
  Divide4/1 -> Goto29/1  "vel_outflow_omega"
  Gain10/1 -> Divide3/4
  Square13/1 -> Product20/5
  Product22/1 -> Square13/1
  From76/1 -> Gain11/1
  From73/1 -> Square12/1
  From75/1 -> Gain10/1
  Gain13/1 -> Square14/1
  Product21/1 -> Divide4/2  "outlet_area"
  Gain12/1 -> Product20/4
  From74/1 -> Divide3/3
  Square12/1 -> Product21/2
  outflow_tube_length_m/1 -> Product20/2
  Gain11/1 -> Product20/3
  Gain9/1 -> Saturation5/1
  Constant33/1 -> Product21/1
  Constant32/1 -> Divide3/1
  [x_HP] -> Divide6/2
  Saturation/1 -> Terminator3/1  "k_HP"
  Divide6/1 -> Saturation/1
  Pa_to_PSI1/1 -> Terminator6/1  "TG_reaction_pressure_PSI"
  Ramp/1 -> ?  "alpha0"
  Repeating Sequence Interpolated/1 -> ?  "Eb"
  Repeating Sequence Interpolated1/1 -> ?  "L0"
  Repeating Sequence Interpolated2/1 -> ?  "R0"
  Repeating Sequence Interpolated3/1 -> ?  "t_w0"
  [Q] -> Product13/1
  fluid_damping1/1 -> Product13/2
  Ramp2/1 -> ?  "alpha0"
  Product11/1 -> Gain6/1
  Moving Average/1 -> Terminator10/1  "elec_watt_mov_avg"
  Saturation2/1 -> [elec_power]
  Integrator/1 -> m3_to_L/1  "acc_volume_m3"
  Gain/1 -> Bias/1
  Bias/1 -> Terminator/1, Gain1/1  "acc_press_PSI"
  m3_to_L/1 -> Gain/1
  Gain1/1 -> [acc_press_Pa]  "acc_press_Pa"
  Add/1 -> Integrator/1
  orifice_area/1 -> Product/1
  discharge_coeff/1 -> Product/2
  Sqrt2/1 -> Product/3
  Product1/1 -> Sqrt2/1
  const/1 -> Product1/1
  Subtract1/1 -> Product1/2
  [acc_press_Pa] -> Subtract1/1
  From1/1 -> Subtract1/2
  [acc_press_Pa] -> Chart/1(accumulator_press)
  Constant12/1 -> Chart/2(opening_threshold_press)
  Constant13/1 -> Chart/3(closing_threshold_press)
  Product/1 -> Product2/1
  Chart/1(servo_valve_cmd) -> Product2/2  "SV_cmd"
  Product2/1 -> [acc_outflow]  "acc_outflow_m3_s"
  [acc_outflow] -> Add/2
  [acc_outflow] -> turbine_generator_v0/1
  [acc_press_Pa] -> Add8/1
